simulink model "sd_filter_tb"  (R2020b)
settings: Solver=VariableStepAuto  StartTime=0.0  StopTime=t_stop  RelTol=1e-3
values from neighbouring files (symbols this model uses):
  ts = 1/fs    (= 8.85770975057e-08)    [sd_2nd_mod.m]    (also in sd_2nd_mod_top.m; sd_filter_top.m)
settings Model: Creator=Legion  LastModifiedBy=1111293

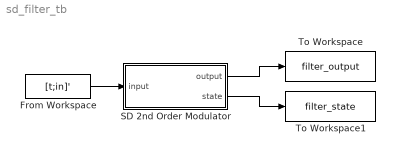
== system sd_filter_tb ==
  From Workspace : FromWorkspace  VariableName=[t;in]'  SampleTime=ts
  SD 2nd Order Modulator : Subsystem
  To Workspace : ToWorkspace  VariableName=filter_output  SaveFormat=Structure With Time  SampleTime=-1
  To Workspace1 : ToWorkspace  VariableName=filter_state  SaveFormat=Structure With Time  SampleTime=-1
  wires:
  From Workspace/1 -> SD 2nd Order Modulator/1(input)
  SD 2nd Order Modulator/1(output) -> To Workspace/1
  SD 2nd Order Modulator/2(state) -> To Workspace1/1

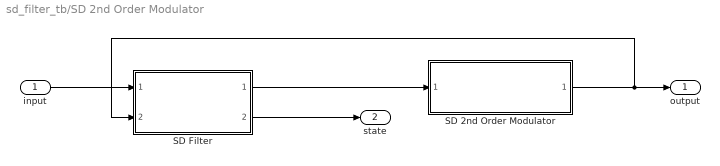
== system sd_filter_tb/SD 2nd Order Modulator ==
  input : Inport
  SD 2nd Order Modulator : Subsystem  ReferencedSubsystem=SD_2nd_Order_Modulator
  SD Filter : Subsystem  ReferencedSubsystem=SD_Filter
  output : Outport
  state : Outport  Port=2
  wires:
  input/1 -> SD Filter/1
  SD Filter/2 -> state/1
  SD Filter/1 -> SD 2nd Order Modulator/1
  SD 2nd Order Modulator/1 -> SD Filter/2, output/1
